simulink model "SF029A_StabyCmp"  (R2013b)
settings: Solver=FixedStepDiscrete  SolverMode=SingleTasking  StartTime=0.0  StopTime=1  FixedStep=0.002  RelTol=1e-3
values from neighbouring files (symbols this model uses):
  ARCHGLBPRM_2MILLISEC_SEC_F32 = DataDict.Constant    [SF029A_StabyCmp_DataDict.m]
  CMPINPLIM_MOTNWTMTR_F32 = DataDict.Constant    [SF029A_StabyCmp_DataDict.m]
  FLTINJ_STABYCMP_ASSICMD = DataDict.Constant    [SF029A_StabyCmp_DataDict.m]
undefined symbols (not defined in the file): StabyCmpNotchFil1Struct, StabyCmpNotchFil2Struct, StabyCmpNotchFil3Struct, StabyCmpNotchFil4Struct
libraries: NxtrMath x5, FixdToFloat x5, FloatToFixd x5, BilnrIntrpnMplX x4, Fil x2, NxtrLim x2, simulink x1, NxtrAbslt x1, LnrIntrpn x1
(part 2 of 2)

== system SF029A_StabyCmp/StabyCmp/StabyCmpPer1/StabiyCmp/Compensator Set 3//4/Compensator 4 ==
  Assist : Inport
  CompFilter_FwdPath : Subsystem
  CompFilter_UpdateSV : Subsystem
  CopyRight2 : Subsystem  Description=|  mask(Copyright Information){none=on}
      | Copyright info block.                                               
      |                                                                     
      | Place copyright information at the top of every subsystem in design.
      mask prompts: none "No parameters"
      mask help: Place copyright information at the top of every subsystem in design.
      mask Display:
      | NxtrConf = 'Nexteer Confidential';
      | 
      | sys = bdroot; %handle for the current model ("system")
      | first = get_param(sys,'Created');
      | if(isempty(first))
      |     first = datestr(now,'yyyy');
      | else
      |     first = first(end-3:end);  %year is last four digits
      | end
      | 
      | last = get_param(sys,'LastModifiedDate');
      | if isempty(last)
      |     last = datestr(now,'yyyy');
      | else
      |     last = last(end-3:end);
      | end
      | 
      | if strcmp(first,last)
      |     fprintf('%s -- Copyright %s Nexteer',NxtrConf,first)
      | else
      |     fprintf('%s -- %s%s- %s Nexteer',NxtrConf,char(169),first,last)
      | end
  Data Store Read : DataStoreRead  Priority=1  DataStoreName=AssiNotch4Fil1  DataStoreElements=AssiNotch4Fil1
  Data Store Read1 : DataStoreRead  Priority=1  DataStoreName=AssiNotch4Fil2  DataStoreElements=AssiNotch4Fil2
  Data Store Write : DataStoreWrite  Priority=2  DataStoreName=AssiNotch4Fil1  DataStoreElements=AssiNotch4Fil1
  Data Store Write1 : DataStoreWrite  Priority=2  DataStoreName=AssiNotch4Fil2  DataStoreElements=AssiNotch4Fil2
  Comp4_Output : Outport
  wires:
  CompFilter_FwdPath/1(CompFilterOut) -> Comp4_Output/1, CompFilter_UpdateSV/2(CompFiltOut)
  CompFilter_UpdateSV/2(CompFiltSV2) -> Data Store Write1/1
  CompFilter_UpdateSV/1(CompFiltSV1) -> Data Store Write/1
  Assist/1 -> CompFilter_FwdPath/1(AssistSumLimit), CompFilter_UpdateSV/1(AsstSumLimit_MtrNm)
  Data Store Read/1 -> CompFilter_FwdPath/2(CompFiltSV1_prev)
  Data Store Read1/1 -> CompFilter_UpdateSV/3(CompFiltSV2_Prev)

== system SF029A_StabyCmp/StabyCmp/StabyCmpPer1/StabiyCmp/Compensator Set 3//4/CopyRight2 ==

== system SF029A_StabyCmp/StabyCmp/StabyCmpPer1/StabiyCmp/Compensator Set 1//2/Compensator 1/CompFilter_FwdPath ==
  AssistSumLimit : Inport
  CompFiltSV1_prev : Inport  Port=2
  B0 : Gain  Gain=B0  RndMeth=Zero
  CopyRight2 : Subsystem  Description=|  mask(Copyright Information){none=on}
      | Copyright info block.                                               
      |                                                                     
      | Place copyright information at the top of every subsystem in design.
      mask prompts: none "No parameters"
      mask help: Place copyright information at the top of every subsystem in design.
      mask Display:
      | NxtrConf = 'Nexteer Confidential';
      | 
      | sys = bdroot; %handle for the current model ("system")
      | first = get_param(sys,'Created');
      | if(isempty(first))
      |     first = datestr(now,'yyyy');
      | else
      |     first = first(end-3:end);  %year is last four digits
      | end
      | 
      | last = get_param(sys,'LastModifiedDate');
      | if isempty(last)
      |     last = datestr(now,'yyyy');
      | else
      |     last = last(end-3:end);
      | end
      | 
      | if strcmp(first,last)
      |     fprintf('%s -- Copyright %s Nexteer',NxtrConf,first)
      | else
      |     fprintf('%s -- %s%s- %s Nexteer',NxtrConf,char(169),first,last)
      | end
  Sum3 : Sum  Inputs=|++  RndMeth=Zero
  CompFilterOut : Outport
  wires:
  AssistSumLimit/1 -> B0/1
  CompFiltSV1_prev/1 -> Sum3/2
  B0/1 -> Sum3/1
  Sum3/1 -> CompFilterOut/1

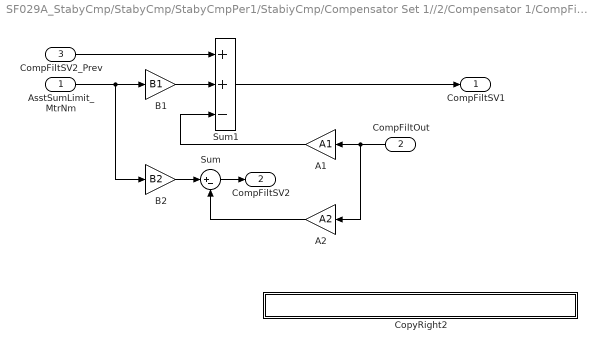
== system SF029A_StabyCmp/StabyCmp/StabyCmpPer1/StabiyCmp/Compensator Set 1//2/Compensator 1/CompFilter_UpdateSV ==
  AsstSumLimit_MtrNm : Inport
  CompFiltOut : Inport  Port=2
  CompFiltSV2_Prev : Inport  Port=3
  A1 : Gain  Gain=A1  RndMeth=Zero
  A2 : Gain  Gain=A2  RndMeth=Zero
  B1 : Gain  Gain=B1  RndMeth=Zero
  B2 : Gain  Gain=B2  RndMeth=Zero
  CopyRight2 : Subsystem  Description=|  mask(Copyright Information){none=on}
      | Copyright info block.                                               
      |                                                                     
      | Place copyright information at the top of every subsystem in design.
      mask prompts: none "No parameters"
      mask help: Place copyright information at the top of every subsystem in design.
      mask Display:
      | NxtrConf = 'Nexteer Confidential';
      | 
      | sys = bdroot; %handle for the current model ("system")
      | first = get_param(sys,'Created');
      | if(isempty(first))
      |     first = datestr(now,'yyyy');
      | else
      |     first = first(end-3:end);  %year is last four digits
      | end
      | 
      | last = get_param(sys,'LastModifiedDate');
      | if isempty(last)
      |     last = datestr(now,'yyyy');
      | else
      |     last = last(end-3:end);
      | end
      | 
      | if strcmp(first,last)
      |     fprintf('%s -- Copyright %s Nexteer',NxtrConf,first)
      | else
      |     fprintf('%s -- %s%s- %s Nexteer',NxtrConf,char(169),first,last)
      | end
  Sum : Sum  Inputs=|+-  RndMeth=Zero
  Sum1 : Sum  Inputs=++-  RndMeth=Zero
  CompFiltSV1 : Outport
  CompFiltSV2 : Outport  Port=2
  wires:
  CompFiltOut/1 -> A2/1, A1/1
  A1/1 -> Sum1/3
  A2/1 -> Sum/2
  Sum1/1 -> CompFiltSV1/1
  B1/1 -> Sum1/2
  CompFiltSV2_Prev/1 -> Sum1/1
  Sum/1 -> CompFiltSV2/1
  B2/1 -> Sum/1
  AsstSumLimit_MtrNm/1 -> B1/1, B2/1

== system SF029A_StabyCmp/StabyCmp/StabyCmpPer1/StabiyCmp/Compensator Set 1//2/Compensator 1/CopyRight2 ==

== system SF029A_StabyCmp/StabyCmp/StabyCmpPer1/StabiyCmp/Compensator Set 1//2/Compensator 2/CompFilter_FwdPath ==
  AssistSumLimit : Inport
  CompFiltSV1_prev : Inport  Port=2
  B0 : Gain  Gain=B0  RndMeth=Zero
  CopyRight2 : Subsystem  Description=|  mask(Copyright Information){none=on}
      | Copyright info block.                                               
      |                                                                     
      | Place copyright information at the top of every subsystem in design.
      mask prompts: none "No parameters"
      mask help: Place copyright information at the top of every subsystem in design.
      mask Display:
      | NxtrConf = 'Nexteer Confidential';
      | 
      | sys = bdroot; %handle for the current model ("system")
      | first = get_param(sys,'Created');
      | if(isempty(first))
      |     first = datestr(now,'yyyy');
      | else
      |     first = first(end-3:end);  %year is last four digits
      | end
      | 
      | last = get_param(sys,'LastModifiedDate');
      | if isempty(last)
      |     last = datestr(now,'yyyy');
      | else
      |     last = last(end-3:end);
      | end
      | 
      | if strcmp(first,last)
      |     fprintf('%s -- Copyright %s Nexteer',NxtrConf,first)
      | else
      |     fprintf('%s -- %s%s- %s Nexteer',NxtrConf,char(169),first,last)
      | end
  Sum3 : Sum  Inputs=|++  RndMeth=Zero
  CompFilterOut : Outport
  wires:
  Sum3/1 -> CompFilterOut/1
  B0/1 -> Sum3/1
  CompFiltSV1_prev/1 -> Sum3/2
  AssistSumLimit/1 -> B0/1

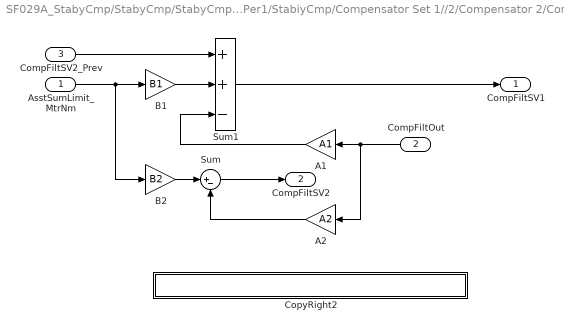
== system SF029A_StabyCmp/StabyCmp/StabyCmpPer1/StabiyCmp/Compensator Set 1//2/Compensator 2/CompFilter_UpdateSV ==
  AsstSumLimit_MtrNm : Inport
  CompFiltOut : Inport  Port=2
  CompFiltSV2_Prev : Inport  Port=3
  A1 : Gain  Gain=A1  RndMeth=Zero
  A2 : Gain  Gain=A2  RndMeth=Zero
  B1 : Gain  Gain=B1  RndMeth=Zero
  B2 : Gain  Gain=B2  RndMeth=Zero
  CopyRight2 : Subsystem  Description=|  mask(Copyright Information){none=on}
      | Copyright info block.                                               
      |                                                                     
      | Place copyright information at the top of every subsystem in design.
      mask prompts: none "No parameters"
      mask help: Place copyright information at the top of every subsystem in design.
      mask Display:
      | NxtrConf = 'Nexteer Confidential';
      | 
      | sys = bdroot; %handle for the current model ("system")
      | first = get_param(sys,'Created');
      | if(isempty(first))
      |     first = datestr(now,'yyyy');
      | else
      |     first = first(end-3:end);  %year is last four digits
      | end
      | 
      | last = get_param(sys,'LastModifiedDate');
      | if isempty(last)
      |     last = datestr(now,'yyyy');
      | else
      |     last = last(end-3:end);
      | end
      | 
      | if strcmp(first,last)
      |     fprintf('%s -- Copyright %s Nexteer',NxtrConf,first)
      | else
      |     fprintf('%s -- %s%s- %s Nexteer',NxtrConf,char(169),first,last)
      | end
  Sum : Sum  Inputs=|+-  RndMeth=Zero
  Sum1 : Sum  Inputs=++-  RndMeth=Zero
  CompFiltSV1 : Outport
  CompFiltSV2 : Outport  Port=2
  wires:
  AsstSumLimit_MtrNm/1 -> B2/1, B1/1
  B2/1 -> Sum/1
  Sum/1 -> CompFiltSV2/1
  CompFiltSV2_Prev/1 -> Sum1/1
  B1/1 -> Sum1/2
  Sum1/1 -> CompFiltSV1/1
  A2/1 -> Sum/2
  A1/1 -> Sum1/3
  CompFiltOut/1 -> A1/1, A2/1

== system SF029A_StabyCmp/StabyCmp/StabyCmpPer1/StabiyCmp/Compensator Set 1//2/Compensator 2/CopyRight2 ==

== system SF029A_StabyCmp/StabyCmp/StabyCmpPer1/StabiyCmp/Compensator Set 3//4/Compensator 3/CompFilter_FwdPath ==
  AssistSumLimit : Inport
  CompFiltSV1_prev : Inport  Port=2
  B0 : Gain  Gain=B0  RndMeth=Zero
  CopyRight2 : Subsystem  Description=|  mask(Copyright Information){none=on}
      | Copyright info block.                                               
      |                                                                     
      | Place copyright information at the top of every subsystem in design.
      mask prompts: none "No parameters"
      mask help: Place copyright information at the top of every subsystem in design.
      mask Display:
      | NxtrConf = 'Nexteer Confidential';
      | 
      | sys = bdroot; %handle for the current model ("system")
      | first = get_param(sys,'Created');
      | if(isempty(first))
      |     first = datestr(now,'yyyy');
      | else
      |     first = first(end-3:end);  %year is last four digits
      | end
      | 
      | last = get_param(sys,'LastModifiedDate');
      | if isempty(last)
      |     last = datestr(now,'yyyy');
      | else
      |     last = last(end-3:end);
      | end
      | 
      | if strcmp(first,last)
      |     fprintf('%s -- Copyright %s Nexteer',NxtrConf,first)
      | else
      |     fprintf('%s -- %s%s- %s Nexteer',NxtrConf,char(169),first,last)
      | end
  Sum3 : Sum  Inputs=|++  RndMeth=Zero
  CompFilterOut : Outport
  wires:
  Sum3/1 -> CompFilterOut/1
  B0/1 -> Sum3/1
  CompFiltSV1_prev/1 -> Sum3/2
  AssistSumLimit/1 -> B0/1

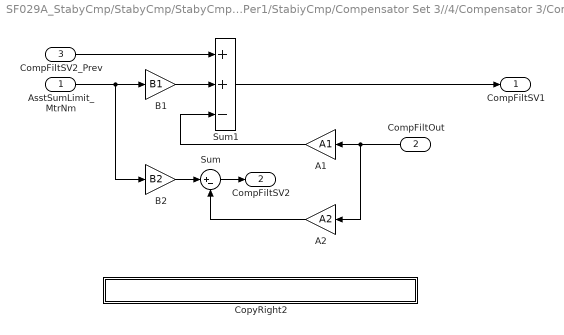
== system SF029A_StabyCmp/StabyCmp/StabyCmpPer1/StabiyCmp/Compensator Set 3//4/Compensator 3/CompFilter_UpdateSV ==
  AsstSumLimit_MtrNm : Inport
  CompFiltOut : Inport  Port=2
  CompFiltSV2_Prev : Inport  Port=3
  A1 : Gain  Gain=A1  RndMeth=Zero
  A2 : Gain  Gain=A2  RndMeth=Zero
  B1 : Gain  Gain=B1  RndMeth=Zero
  B2 : Gain  Gain=B2  RndMeth=Zero
  CopyRight2 : Subsystem  Description=|  mask(Copyright Information){none=on}
      | Copyright info block.                                               
      |                                                                     
      | Place copyright information at the top of every subsystem in design.
      mask prompts: none "No parameters"
      mask help: Place copyright information at the top of every subsystem in design.
      mask Display:
      | NxtrConf = 'Nexteer Confidential';
      | 
      | sys = bdroot; %handle for the current model ("system")
      | first = get_param(sys,'Created');
      | if(isempty(first))
      |     first = datestr(now,'yyyy');
      | else
      |     first = first(end-3:end);  %year is last four digits
      | end
      | 
      | last = get_param(sys,'LastModifiedDate');
      | if isempty(last)
      |     last = datestr(now,'yyyy');
      | else
      |     last = last(end-3:end);
      | end
      | 
      | if strcmp(first,last)
      |     fprintf('%s -- Copyright %s Nexteer',NxtrConf,first)
      | else
      |     fprintf('%s -- %s%s- %s Nexteer',NxtrConf,char(169),first,last)
      | end
  Sum : Sum  Inputs=|+-  RndMeth=Zero
  Sum1 : Sum  Inputs=++-  RndMeth=Zero
  CompFiltSV1 : Outport
  CompFiltSV2 : Outport  Port=2
  wires:
  AsstSumLimit_MtrNm/1 -> B2/1, B1/1
  B2/1 -> Sum/1
  Sum/1 -> CompFiltSV2/1
  CompFiltSV2_Prev/1 -> Sum1/1
  B1/1 -> Sum1/2
  Sum1/1 -> CompFiltSV1/1
  A2/1 -> Sum/2
  A1/1 -> Sum1/3
  CompFiltOut/1 -> A1/1, A2/1

== system SF029A_StabyCmp/StabyCmp/StabyCmpPer1/StabiyCmp/Compensator Set 3//4/Compensator 3/CopyRight2 ==

== system SF029A_StabyCmp/StabyCmp/StabyCmpPer1/StabiyCmp/Compensator Set 3//4/Compensator 4/CompFilter_FwdPath ==
  AssistSumLimit : Inport
  CompFiltSV1_prev : Inport  Port=2
  B0 : Gain  Gain=B0  RndMeth=Zero
  CopyRight2 : Subsystem  Description=|  mask(Copyright Information){none=on}
      | Copyright info block.                                               
      |                                                                     
      | Place copyright information at the top of every subsystem in design.
      mask prompts: none "No parameters"
      mask help: Place copyright information at the top of every subsystem in design.
      mask Display:
      | NxtrConf = 'Nexteer Confidential';
      | 
      | sys = bdroot; %handle for the current model ("system")
      | first = get_param(sys,'Created');
      | if(isempty(first))
      |     first = datestr(now,'yyyy');
      | else
      |     first = first(end-3:end);  %year is last four digits
      | end
      | 
      | last = get_param(sys,'LastModifiedDate');
      | if isempty(last)
      |     last = datestr(now,'yyyy');
      | else
      |     last = last(end-3:end);
      | end
      | 
      | if strcmp(first,last)
      |     fprintf('%s -- Copyright %s Nexteer',NxtrConf,first)
      | else
      |     fprintf('%s -- %s%s- %s Nexteer',NxtrConf,char(169),first,last)
      | end
  Sum3 : Sum  Inputs=|++  RndMeth=Zero
  CompFilterOut : Outport
  wires:
  AssistSumLimit/1 -> B0/1
  CompFiltSV1_prev/1 -> Sum3/2
  B0/1 -> Sum3/1
  Sum3/1 -> CompFilterOut/1

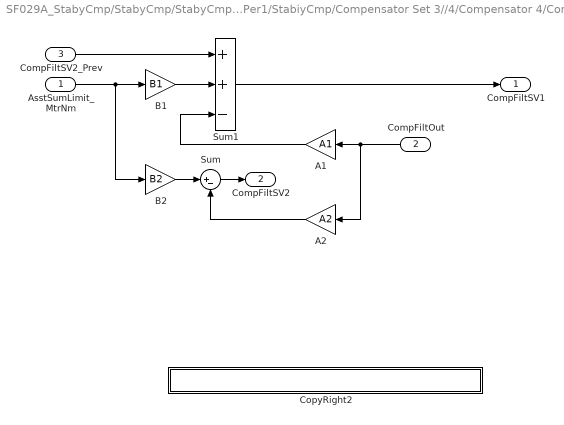
== system SF029A_StabyCmp/StabyCmp/StabyCmpPer1/StabiyCmp/Compensator Set 3//4/Compensator 4/CompFilter_UpdateSV ==
  AsstSumLimit_MtrNm : Inport
  CompFiltOut : Inport  Port=2
  CompFiltSV2_Prev : Inport  Port=3
  A1 : Gain  Gain=A1  RndMeth=Zero
  A2 : Gain  Gain=A2  RndMeth=Zero
  B1 : Gain  Gain=B1  RndMeth=Zero
  B2 : Gain  Gain=B2  RndMeth=Zero
  CopyRight2 : Subsystem  Description=|  mask(Copyright Information){none=on}
      | Copyright info block.                                               
      |                                                                     
      | Place copyright information at the top of every subsystem in design.
      mask prompts: none "No parameters"
      mask help: Place copyright information at the top of every subsystem in design.
      mask Display:
      | NxtrConf = 'Nexteer Confidential';
      | 
      | sys = bdroot; %handle for the current model ("system")
      | first = get_param(sys,'Created');
      | if(isempty(first))
      |     first = datestr(now,'yyyy');
      | else
      |     first = first(end-3:end);  %year is last four digits
      | end
      | 
      | last = get_param(sys,'LastModifiedDate');
      | if isempty(last)
      |     last = datestr(now,'yyyy');
      | else
      |     last = last(end-3:end);
      | end
      | 
      | if strcmp(first,last)
      |     fprintf('%s -- Copyright %s Nexteer',NxtrConf,first)
      | else
      |     fprintf('%s -- %s%s- %s Nexteer',NxtrConf,char(169),first,last)
      | end
  Sum : Sum  Inputs=|+-  RndMeth=Zero
  Sum1 : Sum  Inputs=++-  RndMeth=Zero
  CompFiltSV1 : Outport
  CompFiltSV2 : Outport  Port=2
  wires:
  CompFiltOut/1 -> A2/1, A1/1
  A1/1 -> Sum1/3
  A2/1 -> Sum/2
  Sum1/1 -> CompFiltSV1/1
  B1/1 -> Sum1/2
  CompFiltSV2_Prev/1 -> Sum1/1
  Sum/1 -> CompFiltSV2/1
  B2/1 -> Sum/1
  AsstSumLimit_MtrNm/1 -> B1/1, B2/1

== system SF029A_StabyCmp/StabyCmp/StabyCmpPer1/StabiyCmp/Compensator Set 3//4/Compensator 4/CopyRight2 ==

== system SF029A_StabyCmp/StabyCmp/StabyCmpPer1/StabiyCmp/Compensator Set 1//2/Compensator 1/CompFilter_FwdPath/CopyRight2 ==

== system SF029A_StabyCmp/StabyCmp/StabyCmpPer1/StabiyCmp/Compensator Set 1//2/Compensator 1/CompFilter_UpdateSV/CopyRight2 ==

== system SF029A_StabyCmp/StabyCmp/StabyCmpPer1/StabiyCmp/Compensator Set 1//2/Compensator 2/CompFilter_FwdPath/CopyRight2 ==

== system SF029A_StabyCmp/StabyCmp/StabyCmpPer1/StabiyCmp/Compensator Set 1//2/Compensator 2/CompFilter_UpdateSV/CopyRight2 ==

== system SF029A_StabyCmp/StabyCmp/StabyCmpPer1/StabiyCmp/Compensator Set 3//4/Compensator 3/CompFilter_FwdPath/CopyRight2 ==

== system SF029A_StabyCmp/StabyCmp/StabyCmpPer1/StabiyCmp/Compensator Set 3//4/Compensator 3/CompFilter_UpdateSV/CopyRight2 ==

== system SF029A_StabyCmp/StabyCmp/StabyCmpPer1/StabiyCmp/Compensator Set 3//4/Compensator 4/CompFilter_FwdPath/CopyRight2 ==

== system SF029A_StabyCmp/StabyCmp/StabyCmpPer1/StabiyCmp/Compensator Set 3//4/Compensator 4/CompFilter_UpdateSV/CopyRight2 ==
